simulink model "system_model"  (R2021a)
settings: Solver=VariableStepAuto  StartTime=0.0  StopTime=SimEndTime  RelTol=1e-3
undefined symbols (not defined in the file): Iout_ref
libraries: SignalEditorBlockLib x1, simulink x1
settings Model: DataDictionary=system_data.sldd  Creator=tshintai  LastModifiedBy=tshintai
settings SolverCC: AlgebraicLoopSolver=TrustRegion
settings OptimizationCC: DefaultParameterBehavior=Inlined  EnhancedBackFolding=on  PassReuseOutputArgsAs=Individual arguments  ZeroExternalMemoryAtStartup=off  ZeroInternalMemoryAtStartup=off  OptimizeBlockOrder=speed  DifferentSizesBufferReuse=on  OptimizationCustomize=off  EfficientTunableParamExpr=on
settings DebuggingCC: ParameterTunabilityLossMsg=error  SFMachineParentedDataDiag=warning
settings SFSimCC: MATLABDynamicMemAlloc=off
settings RTWCC: SystemTargetFile=ert.tlc  TemplateMakefile=ert_default_tmf  CodeExecutionProfiling=on  CodeProfilingSaveOptions=AllData
settings CodeAppCC: ForceParamTrailComments=on  IgnoreCustomStorageClasses=off  OperatorAnnotations=on  SimulinkDataObjDesc=on  SFDataObjDesc=on  InsertBlockDesc=on
settings ERTTargetCC: TargetLangStandard=C99 (ISO)  GenerateSampleERTMain=on  InlinedParameterPlacement=NonHierarchical  ERTCustomFileTemplate=example_file_process.tlc

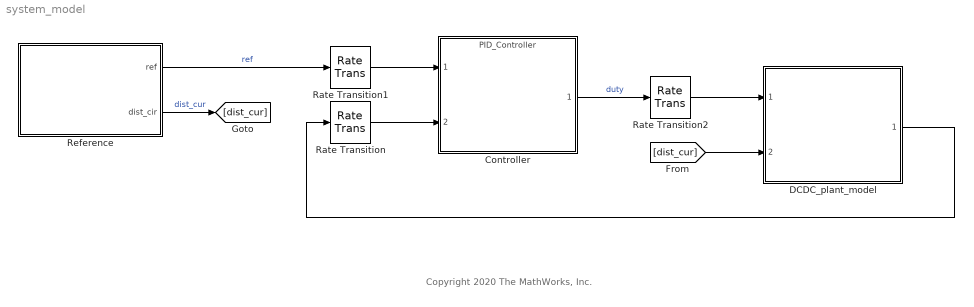
== system system_model ==
  note: Copyright 2020 The MathWorks, Inc.
  Controller : ModelReference  ModelNameDialog=PID_Controller  SimulationMode=Normal  ModelReferenceVersion=2.1
  DCDC_plant_model : Subsystem  ReferencedSubsystem=DCDC_plant_model
  Rate Transition : RateTransition  OutPortSampleTime=TimeStep
  Rate Transition1 : RateTransition  OutPortSampleTime=TimeStep
  Rate Transition2 : RateTransition
  Reference : Subsystem
  wires:
  Controller/1 -> Rate Transition2/1  "duty"
  DCDC_plant_model/1 -> Rate Transition/1
  Reference/1(ref) -> Rate Transition1/1  "ref"
  Rate Transition/1 -> Controller/2
  Rate Transition1/1 -> Controller/1
  Rate Transition2/1 -> DCDC_plant_model/1
  Reference/2(dist_cir) -> [dist_cur]  "dist_cur"
  [dist_cur] -> DCDC_plant_model/2

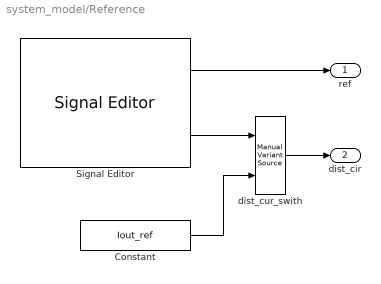
== system system_model/Reference ==
  Constant : Constant  Value=Iout_ref
  Signal Editor : SignalEditorBlockLib/Signal Editor  FileName=ref_signal.mat  ActiveScenario=Step_current_work  ActiveSignal=Vref  IsBus=off  OutputBusObjectStr=Bus: BusObject  SampleTime=0  ZeroCross=off  OutputAfterFinalValue=Holding final value  Unit=inherit  PreserveSignalName=on
  dist_cur_swith : simulink/Signal Routing/Manual Variant Source  NumChoices=2  LabelModeActiveChoice=V_1
  ref : Outport
  dist_cir : Outport  Port=2
  wires:
  Signal Editor/1 -> ref/1
  Signal Editor/2 -> dist_cur_swith/1
  dist_cur_swith/1 -> dist_cir/1
  Constant/1 -> dist_cur_swith/2
